simulink subsystem "global_to_local_waypoint_junho"  (R2022b)
settings: Solver=VariableStepAuto  StartTime=0.0  StopTime=10.0  RelTol=1e-3
settings Model: Creator=USER  LastModifiedBy=User

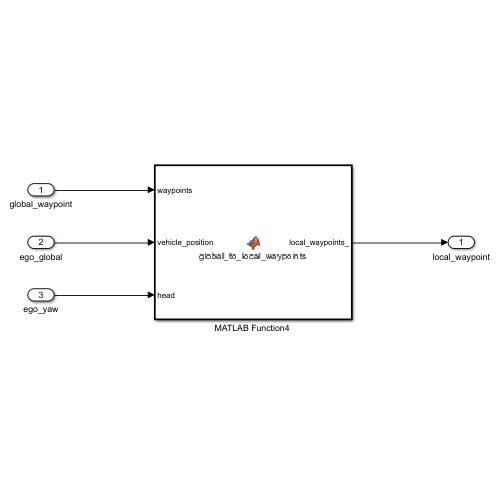
[thumbnail: Simulink's stored preview of the top-level diagram]
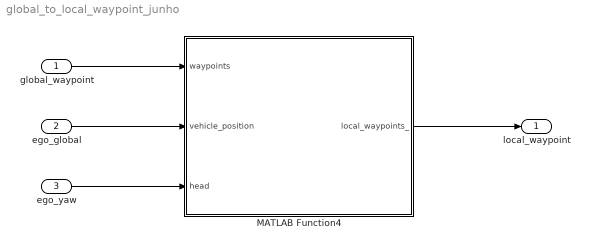
== system global_to_local_waypoint_junho ==
  global_waypoint : Inport
  ego_global : Inport  Port=2
  ego_yaw : Inport  Port=3
  "MATLAB Function4 " : MATLAB Function  TreatAsAtomicUnit=on
  local_waypoint : Outport
  wires:
  "MATLAB Function4 "/1(local_waypoints_) -> local_waypoint/1
  global_waypoint/1 -> "MATLAB Function4 "/1(waypoints)
  ego_global/1 -> "MATLAB Function4 "/2(vehicle_position)
  ego_yaw/1 -> "MATLAB Function4 "/3(head)

== matlab function global_to_local_waypoint_junho/MATLAB Function4  ==
  settings: updateMethod=DISCRETE  sampleTime=0.05
  data: waypoints input; local_waypoints_ output; vehicle_position input; head input
function local_waypoints_ = global_to_local_waypoints_m(waypoints, vehicle_position, head)
   local_waypoints_ = global_to_local_waypoints(waypoints, vehicle_position, head);
end
